simulink model "velocity_PI_control"  (R2021b)
settings: Solver=VariableStepAuto  StartTime=0.0  StopTime=10.0  RelTol=1e-3
undefined symbols (not defined in the file): a, b, ki, kp
settings Model: Creator=DCLab  LastModifiedBy=DCLab

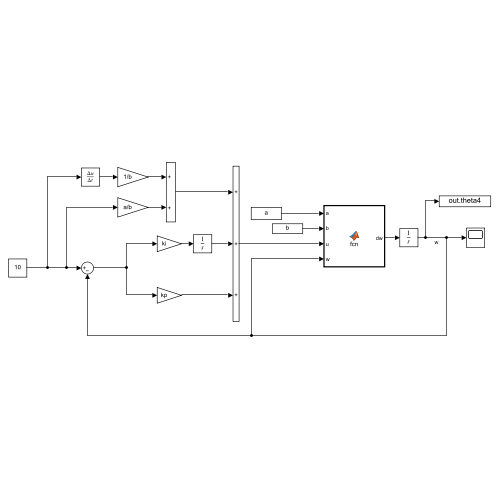
[thumbnail: Simulink's stored preview of the top-level diagram]
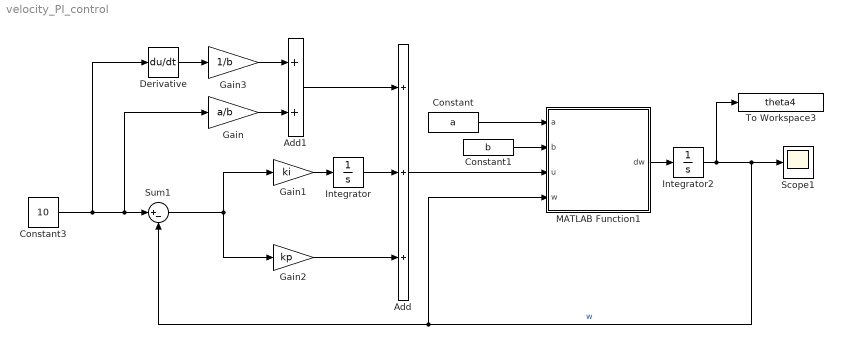
== system velocity_PI_control ==
  Add : Sum  Inputs=+++
  Add1 : Sum
  Constant : Constant  Value=a
  Constant1 : Constant  Value=b
  Constant3 : Constant  Value=10
  Derivative : Derivative
  Gain : Gain  Gain=a/b
  Gain1 : Gain  Gain=ki
  Gain2 : Gain  Gain=kp
  Gain3 : Gain  Gain=1/b
  Integrator : Integrator
  Integrator2 : Integrator
  MATLAB Function1 : MATLAB Function  TreatAsAtomicUnit=on
  Scope1 : Scope
  Sum1 : Sum  Inputs=|+-
  To Workspace3 : ToWorkspace  VariableName=theta4  SampleTime=-1
      settings: Save2DSignal=2-D array (concatenate along first dimension)
  wires:
  MATLAB Function1/1(dw) -> Integrator2/1
  Sum1/1 -> Gain1/1, Gain2/1
  Constant1/1 -> MATLAB Function1/2(b)
  Add/1 -> MATLAB Function1/3(u)
  Integrator2/1 -> To Workspace3/1, Scope1/1, MATLAB Function1/4(w), Sum1/2  "w"
  Gain1/1 -> Integrator/1
  Constant/1 -> MATLAB Function1/1(a)
  Constant3/1 -> Gain/1, Sum1/1, Derivative/1
  Integrator/1 -> Add/2
  Gain2/1 -> Add/3
  Derivative/1 -> Gain3/1
  Gain3/1 -> Add1/1
  Gain/1 -> Add1/2
  Add1/1 -> Add/1

== matlab function velocity_PI_control/MATLAB Function1 ==
  data: a input; dw output; b input; u input; w input
function dw = fcn(a,b,u,w)

dw = -a*w+b*u;
